simulink model "atrias_original"  (R2017a)
settings: Solver=ode45  StartTime=0.0  StopTime=sim_t  RelTol=1e-6  EnableMultiTasking=on
values from neighbouring files (symbols this model uses):
  N = grid_slice*1000    [createGrid.m]
  nm = fn_set_vnmc_params(sm, sample_time)    [kernel_scores_NM_mismatch.m]    (also in main_ATRIAS_cluster.m)
  nmc_BLCtrlPar = nmc.BLCtrlPar    [kernel_scores_NM_mismatch.m]    (also in main_ATRIAS_cluster.m)
  nmc_FPCtrlPar = nmc.FPCtrlPar    [kernel_scores_NM_mismatch.m]    (also in main_ATRIAS_cluster.m)
  nmc_LLCtrlPar = nmc.LLCtrlPar    [kernel_scores_NM_mismatch.m]    (also in main_ATRIAS_cluster.m)
  nmc_StCtrlPar = nmc.StCtrlPar    [kernel_scores_NM_mismatch.m]    (also in main_ATRIAS_cluster.m)
  nmc_SwCtrlPar = nmc.SwCtrlPar    [kernel_scores_NM_mismatch.m]    (also in main_ATRIAS_cluster.m)
  nmc_TrCtrlPar = nmc.TrCtrlPar    [kernel_scores_NM_mismatch.m]    (also in main_ATRIAS_cluster.m)
  nStep_switchCtrl = 10    [main_ATRIAS_cluster.m]
  nStep_thr = 1000    [createSimInitial.m]    (also in main_ATRIAS_cluster.m)
  rc_CtrlPar = [rc.k_placement, rc.T_step, rc.Cd, rc.kpt, rc.kdt, rc.desired_theta, rc.desired_z, rc.kpz, rc.kdz]    [kernel_scores_NM_mismatch.m]    (also in main_ATRIAS_cluster.m)
  sm = fn_set_MechParams(sm)    [kernel_scores_NM_mismatch.m]    (also in main_ATRIAS_cluster.m = fn_set_MechParams(sm,perturb))
  test_VNMC = 1    [createSimInitial.m]    (also in main_ATRIAS_cluster.m = 0)
undefined symbols (not defined in the file or in its folder): delta_phi_max, delta_phi_max_buffer, delta_phi_min, DiscIntNeverNeededParam, Discrete, idc, initial_dx_estimate, initial_dy_estimate, initial_dz_estimate, initial_z_estimate, kd_shin_max, kd_shin_min, kd_splay_max, kd_splay_min, kd_thigh_max, kd_thigh_min, kp_shin_max, kp_shin_min, kp_splay_max, kp_splay_min, kp_thigh_max, kp_thigh_min, mc, min_splay_angle, min_splay_buffer, phi_shin_max, phi_shin_max_buffer, phi_shin_min, phi_shin_min_buffer, phi_thigh_max, phi_thigh_max_buffer, phi_thigh_min, phi_thigh_min_buffer, rad, rc, s, sample_time, sgn, sim_d, t_friction, Time, X, Y, Z
libraries: sm_lib x202, nesl_utility x122, simulink x77, simulink_extras x24, fl_lib x16, mblibv1 x4, ctrlSharedLib x4, commnoisgen2 x1, dspswit3 x1
(part 5 of 17)

== system atrias_original/ATRIAS_sim/Mechanical System Layer/Torso ==
  Acceleration Sensor : sm_lib/Frames and Transforms/Transform Sensor  MeasurementFrame=NonRotatingFollower  SenseAngle=off  SenseAxis=off  SenseAngle1=off  SenseAngle2=off  SenseAngle3=off  SenseQ=off  SenseR=off  SenseOmegaX=off  SenseOmegaY=off  SenseOmegaZ=off  SenseOmega1=off  SenseOmega2=off  SenseOmega3=off  SenseQDot=off  SenseRDot=off  SenseAlphaX=off  SenseAlphaY=off  SenseAlphaZ=off  SenseAlpha1=off  SenseAlpha2=off  SenseAlpha3=off  SenseQDDot=off  SenseRDDot=off  SenseX=off  SenseY=off  SenseZ=off  SenseRad=off  SenseAzim=off  SenseDist=off  SenseInc=off  SenseXDot=off  SenseYDot=off  SenseZDot=off  SenseRadDot=off  SenseAzimDot=off  SenseDistDot=off  SenseIncDot=off  SenseXDDot=on  SenseYDDot=on  SenseZDDot=on  SenseRadDDot=off  SenseAzimDDot=off  SenseDistDDot=off  SenseIncDDot=off
  CS1 to CS2 : sm_lib/Frames and Transforms/Rigid Transform  TranslationMethod=Cartesian  TranslationStandardOffset=0  TranslationLengthUnit=m  TranslationStandardAxis=+Z  TranslationCartesianOffset=sm.torso_12  TranslationROffset=0  TranslationROffsetUnits=m  TranslationZOffset=0  TranslationZOffsetUnits=m  TranslationThetaOffset=0  TranslationThetaOffsetUnits=deg  RotationMethod=None  RotationAngleUnits=deg  RotationStandardAxis=+Z  RotationAngle=0  RotationArbitraryAxis=[0 0 1]  FollAlignAxisA=+X  BaseAlignAxisA=+Y  FollAlignAxisB=+Y  BaseAlignAxisB=+Z  RotationSequenceAxes=FollowerAxes  RotationSequence=XYX  RotationSequenceAngles=[0 0 0]  RotationSequenceAnglesUnits=deg  RotationMatrix=[1 0 0; 0 1 0; 0 0 1]
  Frame Data : Subsystem
  Hip Point to IMU : sm_lib/Frames and Transforms/Rigid Transform  TranslationMethod=Cartesian  TranslationStandardOffset=0  TranslationLengthUnit=m  TranslationStandardAxis=+Z  TranslationCartesianOffset=sm.d_pelvis_to_IMU  TranslationROffset=0  TranslationROffsetUnits=m  TranslationZOffset=0  TranslationZOffsetUnits=m  TranslationThetaOffset=0  TranslationThetaOffsetUnits=deg  RotationMethod=None  RotationAngleUnits=deg  RotationStandardAxis=+Z  RotationAngle=0  RotationArbitraryAxis=[0 0 1]  FollAlignAxisA=+X  BaseAlignAxisA=+Y  FollAlignAxisB=+Y  BaseAlignAxisB=+Z  RotationSequenceAxes=FollowerAxes  RotationSequence=XYX  RotationSequenceAngles=[0 0 0]  RotationSequenceAnglesUnits=deg  RotationMatrix=[1 0 0; 0 1 0; 0 0 1]
  Mux1 : Mux  Inputs=3
  Mux2 : Mux  Inputs=3
  Orientation Sensor : sm_lib/Frames and Transforms/Transform Sensor  MeasurementFrame=Base  SenseAngle=off  SenseAxis=off  SenseAngle1=off  SenseAngle2=off  SenseAngle3=off  SenseQ=off  SenseR=on  SenseOmegaX=off  SenseOmegaY=off  SenseOmegaZ=off  SenseOmega1=off  SenseOmega2=off  SenseOmega3=off  SenseQDot=off  SenseRDot=off  SenseAlphaX=off  SenseAlphaY=off  SenseAlphaZ=off  SenseAlpha1=off  SenseAlpha2=off  SenseAlpha3=off  SenseQDDot=off  SenseRDDot=off  SenseX=off  SenseY=off  SenseZ=off  SenseRad=off  SenseAzim=off  SenseDist=off  SenseInc=off  SenseXDot=off  SenseYDot=off  SenseZDot=off  SenseRadDot=off  SenseAzimDot=off  SenseDistDot=off  SenseIncDot=off  SenseXDDot=off  SenseYDDot=off  SenseZDDot=off  SenseRadDDot=off  SenseAzimDDot=off  SenseDistDDot=off  SenseIncDDot=off
  PS-Simulink Converter{1..3,8} (4 alike) : nesl_utility/PS-Simulink Converter  PhysicalDomain=network_engine_domain  SubClassName=ps_output  LeftPortType=input  RightPortType=output  PseudoPeriodic=off  Frequencies=[]  Unit=1  AffineConversion=off
  Rotation To Euler Angles : MATLAB Function  TreatAsAtomicUnit=on
  Solid : sm_lib/Body Elements/Solid  InertiaType=Custom  Mass=sm.m_torso  MassUnits=kg  CenterOfMass=sm.com_torso  CenterOfMassUnits=m  MomentsOfInertia=sm.i_torso_moments  MomentsOfInertiaUnits=kg*m^2  ProductsOfInertia=sm.i_torso_products  ProductsOfInertiaUnits=kg*m^2  DensityBased=on  Density=1000  DensityUnits=kg/(m^3)  DoExposeReferenceFrame=on  SerializedFrames=<Frames/>  GraphicType=FromGeometry  MarkerShape=Sphere  MarkerSize=10  MarkerSizeUnits=m  GraphicVisPropType=AdvancedVisualProperties  GraphicDiffuseColor=sm.torso_color_d  GraphicSpecularColor=[0.5 0.5 0.5 1.0]  GraphicAmbientColor=[sm.torso_color_d*0.5 1.0]  GraphicEmissiveColor=[0.0 0.0 0.0 1.0]  GraphicShininess=128  GraphicOpacity=1.0  GeometryShape=FromFile  RectangleSize=[1 1]  RectangleSizeUnits=m  BrickDimensions=[1 1 1]  BrickDimensionUnits=m  CylinderRadius=1  CylinderRadiusUnits=m  CylinderLength=1  CylinderLengthUnits=m  SphereRadius=1  SphereRadiusUnits=m  EllipsoidRadii=[1 1 1]  EllipsoidRadiiUnits=m  ExtrusionCrossSection=[1 1; -1 1; -1 -1; 1 -1]  ExtrusionCrossSectionUnits=m  ExtrusionLength=1  ExtrusionLengthUnits=m  PolygonNumSides=3  PolygonOuterRadius=1  PolygonOuterRadiusUnits=m  ExtGeomFileType=STL  ExtGeomFileName=../models/torso.stl  ExtGeomFileUnits=m  RevolutionCrossSection=[1 1; 1 -1; 2 -1; 2 1]  RevolutionCrossSectionUnits=m  RevolutionExtent=Full  RevolutionAngle=180  RevolutionAngleUnits=deg
  World Frame : sm_lib/Frames and Transforms/World Frame
  Yup to Zup Frame : sm_lib/Frames and Transforms/Rigid Transform  TranslationMethod=None  TranslationStandardOffset=0  TranslationLengthUnit=m  TranslationStandardAxis=+Z  TranslationCartesianOffset=0  TranslationROffset=0  TranslationROffsetUnits=m  TranslationZOffset=0  TranslationZOffsetUnits=m  TranslationThetaOffset=0  TranslationThetaOffsetUnits=deg  RotationMethod=AlignedAxes  RotationAngleUnits=deg  RotationStandardAxis=+Z  RotationAngle=0  RotationArbitraryAxis=[0 0 1]  FollAlignAxisA=+Z  BaseAlignAxisA=+Y  FollAlignAxisB=+X  BaseAlignAxisB=+X  RotationSequenceAxes=FollowerAxes  RotationSequence=XYX  RotationSequenceAngles=[0 0 0]  RotationSequenceAnglesUnits=deg  RotationMatrix=[1 0 0; 0 1 0; 0 0 1]
  CS1 : PMIOPort  Port=1  Side=Right
  CS2 : PMIOPort  Port=2  Side=Left
  CS3 : PMIOPort  Port=3  Side=Left
  IMU XYZ Accelerations [m/s^2] x3 : Outport
  IMU Orientation [rad x3] : Outport  Port=2
  wires:
  PS-Simulink Converter8/1 -> Mux1/1
  PS-Simulink Converter1/1 -> Mux1/2
  PS-Simulink Converter2/1 -> Mux1/3
  Mux1/1 -> IMU XYZ Accelerations [m/s^2] x3/1
  PS-Simulink Converter3/1 -> Rotation To Euler Angles/1(R)
  Rotation To Euler Angles/1(roll) -> Mux2/1
  Mux2/1 -> IMU Orientation [rad x3]/1
  Rotation To Euler Angles/3(yaw) -> Mux2/3
  Rotation To Euler Angles/2(pitch) -> Mux2/2
  connections:
  CS1 to CS2/LConn1 -- Frame Data/LConn1 -- CS1/RConn1 -- Solid/RConn1
  CS3/RConn1 -- CS2/RConn1 -- Hip Point to IMU/LConn1 -- CS1 to CS2/RConn1
  Orientation Sensor/RConn1 -- Acceleration Sensor/RConn1 -- Yup to Zup Frame/RConn1
  Hip Point to IMU/RConn1 -- Yup to Zup Frame/LConn1
  Acceleration Sensor/LConn1 -- World Frame/RConn1 -- Orientation Sensor/LConn1
  PS-Simulink Converter3/LConn1 -- Orientation Sensor/RConn2
  Acceleration Sensor/RConn2 -- PS-Simulink Converter8/LConn1
  Acceleration Sensor/RConn3 -- PS-Simulink Converter1/LConn1
  PS-Simulink Converter2/LConn1 -- Acceleration Sensor/RConn4

== system atrias_original/ATRIAS_sim/Mechanical System Layer/Winch ==
  note: Cable cannot push
  Compare To Constant1 : simulink/Logic and Bit Operations/Compare To Constant  relop===  const=-1  OutDataTypeStr=boolean  ZeroCross=off
  Constant1 : Constant  Value=sm.initial_winch_angle
  Constant2 : Constant  Value=0
  Desired Roll Velocity : Constant  Value=0
  Gain2 : Gain  Gain=sm.kp_winch
  Gain3 : Gain  Gain=sm.kd_winch
  PS-Simulink Converter : nesl_utility/PS-Simulink Converter  PhysicalDomain=network_engine_domain  SubClassName=ps_output  LeftPortType=input  RightPortType=output  PseudoPeriodic=off  Frequencies=[]  Unit=1  AffineConversion=off
  PS-Simulink Converter1 : nesl_utility/PS-Simulink Converter  PhysicalDomain=network_engine_domain  SubClassName=ps_output  LeftPortType=input  RightPortType=output  PseudoPeriodic=off  Frequencies=[]  Unit=1  AffineConversion=off
  Pitch Frame : sm_lib/Frames and Transforms/Rigid Transform  TranslationMethod=None  TranslationStandardOffset=0  TranslationLengthUnit=m  TranslationStandardAxis=+Z  TranslationCartesianOffset=[0 0 0]  TranslationROffset=0  TranslationROffsetUnits=m  TranslationZOffset=0  TranslationZOffsetUnits=m  TranslationThetaOffset=0  TranslationThetaOffsetUnits=deg  RotationMethod=AlignedAxes  RotationAngleUnits=rad  RotationStandardAxis=+Z  RotationAngle=0  RotationArbitraryAxis=[1 0 0]  FollAlignAxisA=-Z  BaseAlignAxisA=+X  FollAlignAxisB=+Y  BaseAlignAxisB=+Y  RotationSequenceAxes=FollowerAxes  RotationSequence=XYX  RotationSequenceAngles=[0 0 0]  RotationSequenceAnglesUnits=deg  RotationMatrix=[1 0 0; 0 1 0; 0 0 1]
  Roll Frame : sm_lib/Frames and Transforms/Rigid Transform  TranslationMethod=None  TranslationStandardOffset=0  TranslationLengthUnit=m  TranslationStandardAxis=+Z  TranslationCartesianOffset=[0 0 0]  TranslationROffset=0  TranslationROffsetUnits=m  TranslationZOffset=0  TranslationZOffsetUnits=m  TranslationThetaOffset=0  TranslationThetaOffsetUnits=deg  RotationMethod=AlignedAxes  RotationAngleUnits=rad  RotationStandardAxis=+Z  RotationAngle=0  RotationArbitraryAxis=[1 0 0]  FollAlignAxisA=+X  BaseAlignAxisA=-Z  FollAlignAxisB=+Y  BaseAlignAxisB=+Y  RotationSequenceAxes=FollowerAxes  RotationSequence=XYX  RotationSequenceAngles=[0 0 0]  RotationSequenceAnglesUnits=deg  RotationMatrix=[1 0 0; 0 1 0; 0 0 1]
  Roll Joint : sm_lib/Joints/Revolute Joint  SenseConstraintForce=off  SenseConstraintForceX=off  SenseConstraintForceY=off  SenseConstraintForceZ=off  SenseConstraintTorque=off  SenseConstraintTorqueX=off  SenseConstraintTorqueY=off  SenseConstraintTorqueZ=off  SenseTotalForce=off  SenseTotalForceX=off  SenseTotalForceY=off  SenseTotalForceZ=off  SenseTotalTorque=off  SenseTotalTorqueX=off  SenseTotalTorqueY=off  SenseTotalTorqueZ=off  CompositeWrenchDir=FollowerOnBase  CompositeWrenchFrame=BaseFrame  EquilibriumPosition=0  EquilibriumPositionUnits=deg  SpringStiffness=0  SpringStiffnessUnits=N*m/deg  DampingCoefficient=0  DampingCoefficientUnits=N*m/(deg/s)  TorqueActuationMode=InputTorque  MotionActuationMode=ComputedMotion  SensePosition=on  SenseVelocity=on  SenseAcceleration=off  SenseTorqueForce=off  PositionTargetSpecify=on  PositionTargetPriority=High  PositionTargetValue=sm.initial_boom_roll  PositionTargetValueUnits=rad  VelocityTargetSpecify=off  VelocityTargetPriority=High  VelocityTargetValue=0  VelocityTargetValueUnits=deg/s
  Sign1 : Signum  ZeroCross=off
  Simulink-PS Converter : nesl_utility/Simulink-PS Converter  PhysicalDomain=network_engine_domain  SubClassName=ps_input  LeftPortType=input  RightPortType=output  PseudoPeriodic=off  Frequencies=[]  NoiseDistribution=none  NoiseParameters=[]  Unit=1  AffineConversion=off  FilteringAndDerivatives=zero  SimscapeFilterOrder=1  InputFilterTimeConstant=0.001  UdotUserProvided=1
  Sum : Sum  Inputs=+-|
  Sum1 : Sum  Inputs=+|+
  Sum3 : Sum  Inputs=+-|
  Switch : Switch  Threshold=1
  Boom : PMIOPort  Port=1  Side=Right
  Yaw Shaft : PMIOPort  Port=2  Side=Right
  Boom Roll [rad] : Outport
  wires:
  Sum/1 -> Gain2/1
  Sum1/1 -> Switch/3, Sign1/1
  Sign1/1 -> Compare To Constant1/1
  Constant2/1 -> Switch/1
  Compare To Constant1/1 -> Switch/2
  Switch/1 -> Simulink-PS Converter/1
  PS-Simulink Converter/1 -> Boom Roll [rad]/1, Sum/2
  PS-Simulink Converter1/1 -> Sum3/2
  Desired Roll Velocity/1 -> Sum3/1
  Sum3/1 -> Gain3/1
  Gain2/1 -> Sum1/1
  Gain3/1 -> Sum1/2
  Constant1/1 -> Sum/1
  connections:
  Roll Frame/RConn1 -- Roll Joint/LConn1
  Roll Frame/LConn1 -- Yaw Shaft/RConn1
  Boom/RConn1 -- Pitch Frame/RConn1
  Pitch Frame/LConn1 -- Roll Joint/RConn1
  Roll Joint/LConn2 -- Simulink-PS Converter/RConn1
  PS-Simulink Converter/LConn1 -- Roll Joint/RConn2
  PS-Simulink Converter1/LConn1 -- Roll Joint/RConn3

== system atrias_original/ATRIAS_sim/Mechanical System Layer/Yaw Joint ==
  PS-Simulink Converter3 : nesl_utility/PS-Simulink Converter  PhysicalDomain=network_engine_domain  SubClassName=ps_output  LeftPortType=input  RightPortType=output  PseudoPeriodic=off  Frequencies=[]  Unit=1  AffineConversion=off
  Roll Frame : sm_lib/Frames and Transforms/Rigid Transform  TranslationMethod=None  TranslationStandardOffset=0  TranslationLengthUnit=m  TranslationStandardAxis=+Z  TranslationCartesianOffset=[0 0 0]  TranslationROffset=0  TranslationROffsetUnits=m  TranslationZOffset=0  TranslationZOffsetUnits=m  TranslationThetaOffset=0  TranslationThetaOffsetUnits=deg  RotationMethod=AlignedAxes  RotationAngleUnits=rad  RotationStandardAxis=+Z  RotationAngle=0  RotationArbitraryAxis=[1 0 0]  FollAlignAxisA=+Z  BaseAlignAxisA=+Y  FollAlignAxisB=+X  BaseAlignAxisB=+X  RotationSequenceAxes=FollowerAxes  RotationSequence=XYX  RotationSequenceAngles=[0 0 0]  RotationSequenceAnglesUnits=deg  RotationMatrix=[1 0 0; 0 1 0; 0 0 1]
  Yaw Frame : sm_lib/Frames and Transforms/Rigid Transform  TranslationMethod=None  TranslationStandardOffset=0  TranslationLengthUnit=m  TranslationStandardAxis=+Z  TranslationCartesianOffset=[0 0 0]  TranslationROffset=0  TranslationROffsetUnits=m  TranslationZOffset=0  TranslationZOffsetUnits=m  TranslationThetaOffset=0  TranslationThetaOffsetUnits=deg  RotationMethod=AlignedAxes  RotationAngleUnits=rad  RotationStandardAxis=+Z  RotationAngle=0  RotationArbitraryAxis=[1 0 0]  FollAlignAxisA=+Y  BaseAlignAxisA=+Z  FollAlignAxisB=+X  BaseAlignAxisB=+X  RotationSequenceAxes=FollowerAxes  RotationSequence=XYX  RotationSequenceAngles=[0 0 0]  RotationSequenceAnglesUnits=deg  RotationMatrix=[1 0 0; 0 1 0; 0 0 1]
  Yaw Joint : sm_lib/Joints/Revolute Joint  SenseConstraintForce=off  SenseConstraintForceX=off  SenseConstraintForceY=off  SenseConstraintForceZ=off  SenseConstraintTorque=off  SenseConstraintTorqueX=off  SenseConstraintTorqueY=off  SenseConstraintTorqueZ=off  SenseTotalForce=off  SenseTotalForceX=off  SenseTotalForceY=off  SenseTotalForceZ=off  SenseTotalTorque=off  SenseTotalTorqueX=off  SenseTotalTorqueY=off  SenseTotalTorqueZ=off  CompositeWrenchDir=FollowerOnBase  CompositeWrenchFrame=BaseFrame  EquilibriumPosition=0  EquilibriumPositionUnits=deg  SpringStiffness=0  SpringStiffnessUnits=N*m/deg  DampingCoefficient=0  DampingCoefficientUnits=N*m/(deg/s)  TorqueActuationMode=NoTorque  MotionActuationMode=ComputedMotion  SensePosition=on  SenseVelocity=off  SenseAcceleration=off  SenseTorqueForce=off  PositionTargetSpecify=on  PositionTargetPriority=High  PositionTargetValue=sm.initial_boom_yaw  PositionTargetValueUnits=rad  VelocityTargetSpecify=on  VelocityTargetPriority=High  VelocityTargetValue=sm.initial_boom_yaw_velocity  VelocityTargetValueUnits=rad/s
  Yaw Shaft : PMIOPort  Port=1  Side=Right
  Base : PMIOPort  Port=2  Side=Left
  Yaw [rad] : Outport
  wires:
  PS-Simulink Converter3/1 -> Yaw [rad]/1
  connections:
  Yaw Frame/LConn1 -- Base/RConn1
  Yaw Joint/LConn1 -- Yaw Frame/RConn1
  Roll Frame/LConn1 -- Yaw Joint/RConn1
  Roll Frame/RConn1 -- Yaw Shaft/RConn1
  PS-Simulink Converter3/LConn1 -- Yaw Joint/RConn2

== system atrias_original/ATRIAS_sim/Mechanical System Layer/Yaw Shaft ==
  CS1 to CS2 : sm_lib/Frames and Transforms/Rigid Transform  TranslationMethod=Cartesian  TranslationStandardOffset=0  TranslationLengthUnit=m  TranslationStandardAxis=+Z  TranslationCartesianOffset=sm.yshaft_12  TranslationROffset=0  TranslationROffsetUnits=m  TranslationZOffset=0  TranslationZOffsetUnits=m  TranslationThetaOffset=0  TranslationThetaOffsetUnits=deg  RotationMethod=None  RotationAngleUnits=deg  RotationStandardAxis=+Z  RotationAngle=0  RotationArbitraryAxis=[0 0 1]  FollAlignAxisA=+X  BaseAlignAxisA=+Y  FollAlignAxisB=+Y  BaseAlignAxisB=+Z  RotationSequenceAxes=FollowerAxes  RotationSequence=XYX  RotationSequenceAngles=[0 0 0]  RotationSequenceAnglesUnits=deg  RotationMatrix=[1 0 0; 0 1 0; 0 0 1]
  External Boom Camera : sm_lib/Frames and Transforms/Rigid Transform  TranslationMethod=Cartesian  TranslationStandardOffset=0  TranslationLengthUnit=m  TranslationStandardAxis=+Z  TranslationCartesianOffset=[0 0 -4.5]  TranslationROffset=0  TranslationROffsetUnits=m  TranslationZOffset=0  TranslationZOffsetUnits=m  TranslationThetaOffset=0  TranslationThetaOffsetUnits=deg  RotationMethod=None  RotationAngleUnits=deg  RotationStandardAxis=+Z  RotationAngle=0  RotationArbitraryAxis=[0 0 1]  FollAlignAxisA=+X  BaseAlignAxisA=+Y  FollAlignAxisB=+Y  BaseAlignAxisB=+Z  RotationSequenceAxes=FollowerAxes  RotationSequence=XYX  RotationSequenceAngles=[0 0 0]  RotationSequenceAnglesUnits=deg  RotationMatrix=[1 0 0; 0 1 0; 0 0 1]
  Frame Data : Subsystem
  Solid : sm_lib/Body Elements/Solid  InertiaType=Custom  Mass=sm.m_yshaft  MassUnits=kg  CenterOfMass=sm.com_yshaft  CenterOfMassUnits=m  MomentsOfInertia=sm.i_yshaft_moments  MomentsOfInertiaUnits=kg*m^2  ProductsOfInertia=sm.i_yshaft_products  ProductsOfInertiaUnits=kg*m^2  DensityBased=on  Density=1000  DensityUnits=kg/(m^3)  DoExposeReferenceFrame=on  SerializedFrames=<Frames/>  GraphicType=FromGeometry  MarkerShape=Sphere  MarkerSize=10  MarkerSizeUnits=m  GraphicVisPropType=AdvancedVisualProperties  GraphicDiffuseColor=sm.yshaft_color_d  GraphicSpecularColor=[0.5 0.5 0.5 1.0]  GraphicAmbientColor=[sm.yshaft_color_d*0.5 1.0]  GraphicEmissiveColor=[0.0 0.0 0.0 1.0]  GraphicShininess=128  GraphicOpacity=1.0  GeometryShape=FromFile  RectangleSize=[1 1]  RectangleSizeUnits=m  BrickDimensions=[1 1 1]  BrickDimensionUnits=m  CylinderRadius=1  CylinderRadiusUnits=m  CylinderLength=1  CylinderLengthUnits=m  SphereRadius=1  SphereRadiusUnits=m  EllipsoidRadii=[1 1 1]  EllipsoidRadiiUnits=m  ExtrusionCrossSection=[1 1; -1 1; -1 -1; 1 -1]  ExtrusionCrossSectionUnits=m  ExtrusionLength=1  ExtrusionLengthUnits=m  PolygonNumSides=3  PolygonOuterRadius=1  PolygonOuterRadiusUnits=m  ExtGeomFileType=STL  ExtGeomFileName=../models/boom_yaw.stl  ExtGeomFileUnits=m  RevolutionCrossSection=[1 1; 1 -1; 2 -1; 2 1]  RevolutionCrossSectionUnits=m  RevolutionExtent=Full  RevolutionAngle=180  RevolutionAngleUnits=deg
  CS1 : PMIOPort  Port=1  Side=Left
  CS2 : PMIOPort  Port=2  Side=Right
  connections:
  CS2/RConn1 -- External Boom Camera/LConn1 -- CS1 to CS2/RConn1
  CS1/RConn1 -- CS1 to CS2/LConn1 -- Solid/RConn1 -- Frame Data/LConn1

== system atrias_original/Actuator Control Layer/SEA Controller (Torque)/Desired Torque Derivative ==
  Signal x4 : Inport
  Reset [1/0] x4 : Inport  Port=2
  Demux : Demux
  Demux1 : Demux
  Gain1 : Gain  Gain=1/sample_time
  Logical Operator : Logic  Operator=NOT  AllPortsSameDT=off  OutDataTypeStr=boolean
  Mux : Mux
  Product : Product
  difference : simulink/Discrete/Difference  ICPrevInput=0.0  InputProcessing=Inherited  OutMin=[]  OutMax=[]  OutDataType=fixdt(1, 16)  OutScaling=2^-10  DoSatur=off
  two_pole_filter{,1..3} (4 alike) : DiscreteTransferFcn  Numerator=[mc.A_lpf_dtau 0 0]  Denominator=[1 mc.B1_lpf_dtau mc.B2_lpf_dtau]  ExternalReset=Rising  SampleTime=sample_time
      settings: InputPortMap=u0,r7
  Derivative x4 : Outport
  wires:
  Demux/1 -> two_pole_filter/1
  difference/1 -> Product/1
  Mux/1 -> Derivative x4/1
  Signal x4/1 -> Gain1/1
  Gain1/1 -> difference/1
  Logical Operator/1 -> Product/2
  Reset [1/0] x4/1 -> Demux1/1, Logical Operator/1
  two_pole_filter/1 -> Mux/1
  Product/1 -> Demux/1
  two_pole_filter1/1 -> Mux/2
  two_pole_filter2/1 -> Mux/3
  two_pole_filter3/1 -> Mux/4
  Demux/2 -> two_pole_filter1/1
  Demux/3 -> two_pole_filter2/1
  Demux/4 -> two_pole_filter3/1
  Demux1/1 -> two_pole_filter/2
  Demux1/2 -> two_pole_filter1/2
  Demux1/3 -> two_pole_filter2/2
  Demux1/4 -> two_pole_filter3/2

== system atrias_original/control/Data/Subsystem ==
  In : Inport
  Enable : EnablePort
  Out1 : Outport
  wires:
  In/1 -> Out1/1

== system atrias_original/control/Data/Subsystem1 ==
  In1 : Inport
  Enable : EnablePort
  Out1 : Outport
  wires:
  In1/1 -> Out1/1

== system atrias_original/control/Data/state at switch ==
  xTorso : Inport
  Trigger : TriggerPort  VariantControl=Variant  ZeroCross=off
  To Current Workspace2 : ToWorkspace  VariableName=simout_xTorso_switch  SaveFormat=Structure With Time  SampleTime=-1
      settings: MaxDataPoints=1
  wires:
  xTorso/1 -> To Current Workspace2/1

== system atrias_original/control/RC control/Atrias Swing control ==
  note: Convert to
      | four-bar angles
  note: Position control the
      | individual four bar segments
  X COM from Secondary Foot Desired [m m/s m/s^2] : Inport
  Y COM  from Secondary Foot Desired [m m/s m/s^2] : Inport  Port=2
  Z COM  from Secondary Foot Desired [m m/s m/s^2] : Inport  Port=3
  Secondary Front Gear [rad rad/s] : Inport  Port=4
  Secondary Back Gear [rad rad/s] : Inport  Port=5
  Right or Left Stance [1 or 0] : Inport  Port=6
  Secondary Leg Roll [rad rad/s] : Inport  Port=7
  Secondary Leg Length [m m/s] : Inport  Port=8
  Secondary Leg Angle [rad rad/s] : Inport  Port=9
  Torso Pitch [rad rad/s] : Inport  Port=10
  Torso Roll [rad rad/s] : Inport  Port=11
  Pelvis to COM Position [m] x3 : Inport  Port=12
  Pelvis to COM Velocity [m/s] x3 : Inport  Port=13
  Avoid Hitting Mechanical Limits : MATLAB Function  TreatAsAtomicUnit=on
  Back/Front PD : Subsystem
  "Convert COM Position to Joint Angles + Leg Length " : MATLAB Function  TreatAsAtomicUnit=on
  Demux4 : Demux  Outputs=2
  Demux5 : Demux  Outputs=2
  Demux6 : Demux  Outputs=6
  Mux{3..6,8,11} (6 alike) : Mux  Inputs=2
  Virtual Leg to Four Bar : MATLAB Function  TreatAsAtomicUnit=on
  Back Front Motor Torques [Nm Nm] : Outport
  Desired Swing Beta [rad rad/s] : Outport  Port=2
  wires:
  Virtual Leg to Four Bar/5(dfront) -> Avoid Hitting Mechanical Limits/5(dfront_desired)
  Y COM  from Secondary Foot Desired [m m/s m/s^2]/1 -> "Convert COM Position to Joint Angles + Leg Length "/2(Y_star)
  Mux8/1 -> Demux6/1
  "Convert COM Position to Joint Angles + Leg Length "/1(desired_leg_length) -> Mux8/1
  X COM from Secondary Foot Desired [m m/s m/s^2]/1 -> "Convert COM Position to Joint Angles + Leg Length "/1(X_star)
  Secondary Leg Length [m m/s]/1 -> "Convert COM Position to Joint Angles + Leg Length "/11(leg_length)
  "Convert COM Position to Joint Angles + Leg Length "/3(desired_beta) -> Desired Swing Beta [rad rad/s]/1  "lateral motor angle"
  "Convert COM Position to Joint Angles + Leg Length "/2(desired_alpha) -> Mux8/2
  Secondary Leg Angle [rad rad/s]/1 -> "Convert COM Position to Joint Angles + Leg Length "/9(sagittal_angle)
  Secondary Leg Roll [rad rad/s]/1 -> "Convert COM Position to Joint Angles + Leg Length "/10(lateral_angle)  "swing hip angle (lateral)"
  Right or Left Stance [1 or 0]/1 -> "Convert COM Position to Joint Angles + Leg Length "/4(right_left)
  Torso Roll [rad rad/s]/1 -> "Convert COM Position to Joint Angles + Leg Length "/7(roll)
  Torso Pitch [rad rad/s]/1 -> "Convert COM Position to Joint Angles + Leg Length "/8(pitch)
  Virtual Leg to Four Bar/1(back) -> Avoid Hitting Mechanical Limits/1(back_desired)
  Demux4/2 -> Mux11/2
  Demux6/5 -> Virtual Leg to Four Bar/5(dphi)
  Virtual Leg to Four Bar/4(front) -> Avoid Hitting Mechanical Limits/4(front_desired)
  Demux6/6 -> Virtual Leg to Four Bar/6(ddphi)
  Demux6/3 -> Virtual Leg to Four Bar/3(ddl_leg)
  Demux6/2 -> Virtual Leg to Four Bar/2(dl_leg)
  Virtual Leg to Four Bar/3(ddback) -> Avoid Hitting Mechanical Limits/3(ddback_desired)
  Virtual Leg to Four Bar/6(ddfront) -> Avoid Hitting Mechanical Limits/6(ddfront_desired)
  Mux11/1 -> Back/Front PD/5(Measured Velocity [rad/s] [back front])
  Virtual Leg to Four Bar/2(dback) -> Avoid Hitting Mechanical Limits/2(dback_desired)
  Demux6/4 -> Virtual Leg to Four Bar/4(phi)
  Demux6/1 -> Virtual Leg to Four Bar/1(l_leg)
  Back/Front PD/1(Commanded Torque [Nm] [back front]) -> Back Front Motor Torques [Nm Nm]/1
  Secondary Back Gear [rad rad/s]/1 -> Demux5/1
  Demux5/1 -> Mux6/1
  Z COM  from Secondary Foot Desired [m m/s m/s^2]/1 -> "Convert COM Position to Joint Angles + Leg Length "/3(Z_star)
  Mux4/1 -> Back/Front PD/2(Desired Velocity [rad/s] [back front])
  Secondary Front Gear [rad rad/s]/1 -> Demux4/1
  Demux5/2 -> Mux11/1
  Avoid Hitting Mechanical Limits/3(dback_cmd) -> Mux4/1
  Mux5/1 -> Back/Front PD/3(Desired Acceleration [rad/s^2] [back front])
  Mux3/1 -> Back/Front PD/1(Desired Position [rad] [back front])
  Mux6/1 -> Back/Front PD/4(Measured Position [rad] [back front])
  Avoid Hitting Mechanical Limits/6(ddfront_cmd) -> Mux5/2
  Avoid Hitting Mechanical Limits/5(ddback_cmd) -> Mux5/1
  Avoid Hitting Mechanical Limits/2(front_cmd) -> Mux3/2
  Avoid Hitting Mechanical Limits/4(dfront_cmd) -> Mux4/2
  Avoid Hitting Mechanical Limits/1(back_cmd) -> Mux3/1
  Demux4/1 -> Mux6/2
  Pelvis to COM Position [m] x3/1 -> "Convert COM Position to Joint Angles + Leg Length "/5(com_pelvis_body)
  Pelvis to COM Velocity [m/s] x3/1 -> "Convert COM Position to Joint Angles + Leg Length "/6(dcom_pelvis_body)

== system atrias_original/control/RC control/Enabled Subsystem1 ==
  In1 : Inport
  Enable : EnablePort
  Out1 : Outport
  wires:
  In1/1 -> Out1/1

== system atrias_original/control/RC control/Estimate Angular Accelerations2 ==
  Angular Velocities [rad/s] x3 : Inport
  Enabled : Inport  Port=2
  Detect Change : simulink/Logic and Bit Operations/Detect Change  vinit=0  InputProcessing=Inherited  OutDataTypeStr=boolean
  Difference : simulink/Discrete/Difference  ICPrevInput=0.0  InputProcessing=Inherited  OutMin=[]  OutMax=[]  OutDataType=fixdt(1, 16)  OutScaling=2^-10  DoSatur=off
  Gain : Gain  Gain=1/sample_time
  IMU Two Pole Filter1 : DiscreteTransferFcn  Numerator=[mc.A_lpf_imu 0 0]  Denominator=[1 mc.B1_lpf_imu mc.B2_lpf_imu]  SampleTime=sample_time
  Logical Operator5 : Logic  Operator=NOT  AllPortsSameDT=off  OutDataTypeStr=boolean
  Product : Product
  Angular Accelerations [rad/s^2] x3 : Outport
  wires:
  Enabled/1 -> Detect Change/1
  Logical Operator5/1 -> Product/2
  Angular Velocities [rad/s] x3/1 -> Difference/1
  Gain/1 -> Product/1
  Difference/1 -> Gain/1
  Detect Change/1 -> Logical Operator5/1
  Product/1 -> IMU Two Pole Filter1/1
  IMU Two Pole Filter1/1 -> Angular Accelerations [rad/s^2] x3/1

== system atrias_original/control/RC control/Estimate Angular Accelerations3 ==
  Angular Velocities [rad/s] x2 : Inport
  Enabled : Inport  Port=2
  Detect Change : simulink/Logic and Bit Operations/Detect Change  vinit=0  InputProcessing=Inherited  OutDataTypeStr=boolean
  Difference : simulink/Discrete/Difference  ICPrevInput=0.0  InputProcessing=Inherited  OutMin=[]  OutMax=[]  OutDataType=fixdt(1, 16)  OutScaling=2^-10  DoSatur=off
  Gain : Gain  Gain=1/sample_time
  Lateral Angle Two Pole Filter1 : DiscreteTransferFcn  Numerator=[mc.A_lpf_lateral_angle 0 0]  Denominator=[1 mc.B1_lpf_lateral_angle mc.B2_lpf_lateral_angle]  SampleTime=sample_time
  Logical Operator5 : Logic  Operator=NOT  AllPortsSameDT=off  OutDataTypeStr=boolean
  Product : Product
  Angular Accelerations [rad/s^2] x2 : Outport
  wires:
  Detect Change/1 -> Logical Operator5/1
  Difference/1 -> Gain/1
  Gain/1 -> Product/1
  Angular Velocities [rad/s] x2/1 -> Difference/1
  Logical Operator5/1 -> Product/2
  Enabled/1 -> Detect Change/1
  Product/1 -> Lateral Angle Two Pole Filter1/1
  Lateral Angle Two Pole Filter1/1 -> Angular Accelerations [rad/s^2] x2/1

== system atrias_original/control/RC control/Fz_commanded ==
  measured_z : Inport
  measured_zd : Inport  Port=2
  desired_z : Inport  Port=3
  "Primary Measured Vertical [N}" : Inport  Port=4
  COM XYZ Acceleration [m/s^2] x3 : Inport  Port=5
  kpz : Inport  Port=6
  kdz : Inport  Port=7
  Clamp2 : Saturate  UpperLimit=inf  LowerLimit=0
      settings: AttributesFormatString=Top: %<UpperLimit>\nBottom: %<LowerLimit>
  Clamp3 : Saturate  UpperLimit=inf  LowerLimit=1
      settings: AttributesFormatString=Top: %<UpperLimit>\nBottom: %<LowerLimit>
  Clamp4 : Saturate  UpperLimit=1  LowerLimit=0
      settings: AttributesFormatString=Top: %<UpperLimit>\nBottom: %<LowerLimit>
  Compute Forces1 : Subsystem
  Constant1 : Constant  Commented=on  Value=0.87
  Constant2 : Constant  Commented=on
  Constant3 : Constant
  Constant6 : Constant  Value=mc.m_total_real*mc.g
  Constant7 : Constant  Value=0
  Divide : Product  Inputs=**
  Divide1 : Product  Inputs=*/
  Fcn : Fcn  Expr=1-u
  From82 : From  Commented=on  GotoTag=RightLeft
  Fz : Scope
  Fz Factor : Scope
  Gain8 : Gain  Gain=1/(2*mc.m_total_real*mc.g)
  Mux : Mux  Inputs=2
  Mux35 : Mux  Inputs=2
  Saturation : Saturate  UpperLimit=Inf  LowerLimit=0.2*mc.m_total_real*mc.g
  Selector14 : Selector  InputPortWidth=3  IndexOptions=Index vector (dialog)  Indices=[3]  OutputSizes=1
  Sum1 : Sum  Inputs=|++
  Sum2 : Sum  Inputs=+|+
  Sum3 : Sum  Inputs=+-|
  Sum4 : Sum  Inputs=+++
  Sum6 : Sum  Inputs=+-|
  Switch4 : Switch  Commented=on  Criteria=u2 ~= 0
  multiply : Product  Inputs=**
  multiply1 : Product  Inputs=**
  times : Product  Inputs=**
  times1 : Product  Inputs=**
  z tracking : Scope  NumInputPorts=2
  Fz_commanded : Outport
  wires:
  desired_z/1 -> z tracking/1, Sum3/1
  Saturation/1 -> Mux/2, Fz_commanded/1
  measured_zd/1 -> Sum6/2
  Sum6/1 -> multiply1/1
  Constant7/1 -> Sum6/1
  Sum3/1 -> multiply/1
  measured_z/1 -> z tracking/2, Sum3/2
  Constant6/1 -> Sum4/3
  multiply/1 -> Sum4/1
  multiply1/1 -> Sum4/2
  [GRF_Lz] -> Sum1/1
  [GRF_Rz] -> Sum1/2
  Mux/1 -> Fz/1
  Sum1/1 -> Mux/1
  Divide/1 -> Saturation/1
  Sum4/1 -> Divide/1
  Constant1/1 -> Switch4/3
  Constant2/1 -> Switch4/1
  From82/1 -> Switch4/2
  [GRFfromAccelerometer] -> Selector14/1
  "Primary Measured Vertical [N}"/1 -> Clamp2/1
  Selector14/1 -> Clamp3/1
  Clamp3/1 -> Divide1/2, Gain8/1
  Divide1/1 -> Mux35/1, times/1
  Sum2/1 -> [FzFactor], Mux35/2
  Gain8/1 -> Clamp4/1
  Clamp4/1 -> times/2, Fcn/1
  times/1 -> Sum2/1
  Fcn/1 -> times1/1
  Constant3/1 -> times1/2
  times1/1 -> Sum2/2
  Mux35/1 -> Fz Factor/1
  Clamp2/1 -> Divide1/1
  COM XYZ Acceleration [m/s^2] x3/1 -> Compute Forces1/1(XYZ Acceleration)
  Compute Forces1/1(XYZ Force) -> [GRFfromAccelerometer]
  [FzFactor] -> Divide/2
  kpz/1 -> multiply/2
  kdz/1 -> multiply1/2

== system atrias_original/control/RC control/Inverse Dynamics 2D ==
  Desired Vertical GRF [N] : Inport
  Desired Forward GRF [N] : Inport  Port=2
  Leg Length [m m/s] : Inport  Port=3
  Leg Angle [rad rad/s] : Inport  Port=4
  Torso Pitch [rad rad/s] : Inport  Port=5
  Primary w [m] : Inport  Port=6
  Constant2 : Constant  Value=0
  Demux5 : Demux  Outputs=2
  Leg Force-Torque Distribution : Subsystem
  Spring Torques : Selector  InputPortWidth=7  IndexOptions=Index vector (dialog)  Indices=[6 7]  OutputSizes=1
  target_GRF_inverse_dynamics : MATLAB Function  TreatAsAtomicUnit=on
  Leg Force [N] : Outport
  Leg Torque [Nm] : Outport  Port=2
  wires:
  Desired Vertical GRF [N]/1 -> target_GRF_inverse_dynamics/2(GRFz)
  Desired Forward GRF [N]/1 -> target_GRF_inverse_dynamics/1(GRFx)
  Leg Length [m m/s]/1 -> target_GRF_inverse_dynamics/5(l_leg)
  Constant2/1 -> target_GRF_inverse_dynamics/7(tau_rotor_f), target_GRF_inverse_dynamics/8(tau_rotor_b)
  target_GRF_inverse_dynamics/1(z) -> Spring Torques/1
  Demux5/2 -> Leg Force-Torque Distribution/2(Back Spring Torque [Nm])
  Demux5/1 -> Leg Force-Torque Distribution/1(Front Spring Torque [Nm])
  Spring Torques/1 -> Demux5/1
  Primary w [m]/1 -> Leg Force-Torque Distribution/3(w [m]), target_GRF_inverse_dynamics/6(w)
  Leg Force-Torque Distribution/2(Leg Torque [Nm]) -> Leg Torque [Nm]/1
  Torso Pitch [rad rad/s]/1 -> target_GRF_inverse_dynamics/3(theta)
  Leg Angle [rad rad/s]/1 -> target_GRF_inverse_dynamics/4(phi)
  Leg Force-Torque Distribution/1(Leg Force [N]) -> Leg Force [N]/1

== system atrias_original/control/RC control/Primary Secondary Leg Swap ==
  note: q Order:
      |
      | backJointR
      | backGearR
      | frontJointR
      | frontGearR
      |
      | backJointL
      | backGearL
      | frontJointL
      | frontGearL
      |
      | latR
      | latL
      |
      | boomRoll
      | boomYaw
      | boomPitch
  Entering Stance [1/0] : Inport
  R Leg Angle [rad rad/s] : Inport  Port=2
  R Leg Length [m m/s] : Inport  Port=3
  R Leg w [m] : Inport  Port=4
  R Back Joint [rad rad/s] : Inport  Port=5
  R Back Gear [rad rad/s] : Inport  Port=6
  R Front Joint [rad rad/s] : Inport  Port=7
  R Front Gear [rad rad/s] : Inport  Port=8
  L Leg Angle [rad rad/s] : Inport  Port=9
  L Leg Length [m m/s] : Inport  Port=10
  L Leg w [m] : Inport  Port=11
  L Back Joint [rad rad/s] : Inport  Port=12
  L Back Gear [rad rad/s] : Inport  Port=13
  L Front Joint [rad rad/s] : Inport  Port=14
  L Front Gear [rad rad/s] : Inport  Port=15
  Primary Force/Position Control [1/0] : Inport  Port=16
  Primary Back/Front SEA Torque [Nm Nm] : Inport  Port=17
  Primary Back/Front Motor Torque [Nm Nm] : Inport  Port=18
  Secondary Force/Position Control [1/0] : Inport  Port=19
  Secondary Back/Front SEA Torque [Nm Nm] : Inport  Port=20
  Secondary Back/Front Motor Torque [Nm Nm] : Inport  Port=21
  "Right Leg Roll [rad, rad/s]" : Inport  Port=22
  "Left Leg Roll [rad, rad/s]" : Inport  Port=23
  System Time [s] : Inport  Port=24
  Bus Creator : BusCreator  Inputs=22
  Bus Creator1 : BusCreator  Inputs=22
  Bus Selector : BusSelector  OutputSignals=signal1,signal2,signal3,signal4,signal5,signal6,signal7,signal8,signal9,signal10,signal11,signal12,signal13,signal14,signal15,signal16,signal17,signal18,signal19,signal20,signal21,signal22
  Enabled Subsystem : Subsystem  TreatAsAtomicUnit=on
  Manual Switch : ManualSwitch
  Right Left Primary : Scope  NumInputPorts=2
  Select Leg : Constant  OutDataTypeStr=boolean
  Sum5 : Sum  Inputs=|-+
  Switch6 : Switch  Criteria=u2 ~= 0  OutDataTypeStr=Inherit: Inherit via back propagation  ZeroCross=off
  ToggleRightLeftLeg : MATLAB Function  TreatAsAtomicUnit=on
      settings: MinAlgLoopOccurrences=on
  Unit Delay : UnitDelay  InitialCondition=rc.manual_leg_selection  SampleTime=sample_time
  Right/Left Primary [1/0] : Outport
  Primary Leg Angle [rad rad/s] : Outport  Port=2
  Primary Leg Length [m m/s] : Outport  Port=3
  Primary Leg w [m] : Outport  Port=4
  Primary Back Joint [rad rad/s] : Outport  Port=5
  Primary Back Gear [rad rad/s] : Outport  Port=6
  Primary Front Joint [rad rad/s] : Outport  Port=7
  Primary Front Gear [rad rad/s] : Outport  Port=8
  Secondary Leg Angle [rad rad/s] : Outport  Port=9
  Secondary Leg Length [rad rad/s] : Outport  Port=10
  Secondary Leg w [m] : Outport  Port=11
  Secondary Back Joint [rad rad/s] : Outport  Port=12
  Secondary Back Gear [rad rad/s] : Outport  Port=13
  Secondary Front Joint [rad rad/s] : Outport  Port=14
  Secondary Front Gear [rad rad/s] : Outport  Port=15
  R Force/Position Control [1/0] : Outport  Port=16
  R Back/Front SEA Torque [Nm Nm] : Outport  Port=17
  R Back/Front Motor Torque [Nm Nm] : Outport  Port=18
  L Force/Position Control [1/0] : Outport  Port=19
  L Back/Front SEA Torque [Nm Nm] : Outport  Port=20
  L Back/Front Motor Torque [Nm Nm] : Outport  Port=21
  "Primary Leg Roll [rad, rad/s]" : Outport  Port=22
  "Secondary Leg Roll [rad, rad/s]" : Outport  Port=23
  wires:
  Unit Delay/1 -> ToggleRightLeftLeg/2(previous_right_left)
  ToggleRightLeftLeg/1(right_left) -> Unit Delay/1, Manual Switch/1
  Select Leg/1 -> Manual Switch/2
  R Leg w [m]/1 -> Bus Creator1/10, Bus Creator/3
  R Leg Angle [rad rad/s]/1 -> Bus Creator1/8, Bus Creator/1
  R Leg Length [m m/s]/1 -> Bus Creator1/9, Bus Creator/2
  Bus Creator/1 -> Switch6/1
  Bus Creator1/1 -> Switch6/3
  R Back Joint [rad rad/s]/1 -> Bus Creator1/11, Bus Creator/4
  R Back Gear [rad rad/s]/1 -> Bus Creator1/12, Bus Creator/5
  R Front Joint [rad rad/s]/1 -> Bus Creator1/13, Bus Creator/6
  R Front Gear [rad rad/s]/1 -> Bus Creator1/14, Bus Creator/7
  L Leg Angle [rad rad/s]/1 -> Bus Creator1/1, Bus Creator/8
  L Leg Length [m m/s]/1 -> Bus Creator1/2, Bus Creator/9
  L Leg w [m]/1 -> Bus Creator1/3, Bus Creator/10
  L Back Joint [rad rad/s]/1 -> Bus Creator1/4, Bus Creator/11
  L Back Gear [rad rad/s]/1 -> Bus Creator1/5, Bus Creator/12
  L Front Joint [rad rad/s]/1 -> Bus Creator/13, Bus Creator1/6
  L Front Gear [rad rad/s]/1 -> Bus Creator1/7, Bus Creator/14
  Primary Force/Position Control [1/0]/1 -> Bus Creator1/18, Bus Creator/15
  Primary Back/Front SEA Torque [Nm Nm]/1 -> Bus Creator1/19, Bus Creator/16
  Primary Back/Front Motor Torque [Nm Nm]/1 -> Bus Creator1/20, Bus Creator/17
  Secondary Force/Position Control [1/0]/1 -> Bus Creator1/15, Bus Creator/18
  Secondary Back/Front SEA Torque [Nm Nm]/1 -> Bus Creator1/16, Bus Creator/19
  Secondary Back/Front Motor Torque [Nm Nm]/1 -> Bus Creator1/17, Bus Creator/20
  Switch6/1 -> Bus Selector/1
  Bus Selector/1 -> Primary Leg Angle [rad rad/s]/1  "<signal1>"
  Bus Selector/2 -> Primary Leg Length [m m/s]/1  "<signal2>"
  Bus Selector/3 -> Primary Leg w [m]/1  "<signal3>"
  Bus Selector/4 -> Primary Back Joint [rad rad/s]/1  "<signal4>"
  Bus Selector/5 -> Primary Back Gear [rad rad/s]/1  "<signal5>"
  Bus Selector/6 -> Primary Front Joint [rad rad/s]/1  "<signal6>"
  Bus Selector/7 -> Primary Front Gear [rad rad/s]/1  "<signal7>"
  Bus Selector/8 -> Secondary Leg Angle [rad rad/s]/1  "<signal8>"
  Bus Selector/9 -> Secondary Leg Length [rad rad/s]/1  "<signal9>"
  Bus Selector/10 -> Secondary Leg w [m]/1  "<signal10>"
  Bus Selector/11 -> Secondary Back Joint [rad rad/s]/1  "<signal11>"
  Bus Selector/12 -> Secondary Back Gear [rad rad/s]/1  "<signal12>"
  Bus Selector/13 -> Secondary Front Joint [rad rad/s]/1  "<signal13>"
  Bus Selector/14 -> Secondary Front Gear [rad rad/s]/1  "<signal14>"
  Bus Selector/15 -> R Force/Position Control [1/0]/1  "<signal15>"
  Bus Selector/16 -> R Back/Front SEA Torque [Nm Nm]/1  "<signal16>"
  Bus Selector/17 -> R Back/Front Motor Torque [Nm Nm]/1  "<signal17>"
  Bus Selector/18 -> L Force/Position Control [1/0]/1  "<signal18>"
  Bus Selector/19 -> L Back/Front SEA Torque [Nm Nm]/1  "<signal19>"
  Bus Selector/20 -> L Back/Front Motor Torque [Nm Nm]/1  "<signal20>"
  "Right Leg Roll [rad, rad/s]"/1 -> Bus Creator1/22, Bus Creator/21
  "Left Leg Roll [rad, rad/s]"/1 -> Bus Creator1/21, Bus Creator/22
  Bus Selector/21 -> "Primary Leg Roll [rad, rad/s]"/1  "<signal21>"
  Bus Selector/22 -> "Secondary Leg Roll [rad, rad/s]"/1  "<signal22>"
  Manual Switch/1 -> Right Left Primary/1, Right/Left Primary [1/0]/1, Switch6/2
  System Time [s]/1 -> ToggleRightLeftLeg/3(time_sim), Sum5/2, Enabled Subsystem/1(In1)
  Entering Stance [1/0]/1 -> Enabled Subsystem/Enable, ToggleRightLeftLeg/1(toggle)
  Enabled Subsystem/1(Out1) -> Sum5/1
  Sum5/1 -> Right Left Primary/2

== system atrias_original/control/RC control/Recursive Moving Average ==
  dx [m/s] : Inport
  Delay : Delay  DelayLength=rc.dx_avg_samples  InitialCondition=0  UseCircularBuffer=on  SampleTime=sample_time
  Gain : Gain  Gain=1/(rc.dx_avg_samples)
  Sum : Sum  Inputs=-++
  Unit Delay : UnitDelay  SampleTime=sample_time
  dx_avg [m/s] : Outport
  wires:
  dx [m/s]/1 -> Delay/1, Sum/2
  Sum/1 -> Gain/1, Unit Delay/1
  Delay/1 -> Sum/1
  Gain/1 -> dx_avg [m/s]/1
  Unit Delay/1 -> Sum/3

== system atrias_original/control/RC control/Simbicon leg placcement ==
  Ts [s] : Inport
  dx_des [m/s] : Inport  Port=2
  Foot2CoM : Inport  Port=3
  dx_avg [m/s] : Inport  Port=4
  k_placement : Inport  Port=5
  Cd : Inport  Port=6
  Gain1 : Gain  Gain=0.5
  Mux : Mux  Inputs=2
  Mux1 : Mux  Inputs=2
  Product : Product
  Product1 : Product
  Product2 : Product
  Sum : Sum  Inputs=++-
  Sum2 : Sum  Inputs=-+|
  Ts_saturation : Saturate  UpperLimit=inf  LowerLimit=0.2
      settings: AttributesFormatString=Hi: %<UpperLimit>\nLo: %<LowerLimit>
  d : Scope
  d1 : Scope
  dx : Scope
  dx Saturation : Saturate  UpperLimit=rc.desired_xd  LowerLimit=0
      settings: AttributesFormatString=Hi: %<UpperLimit>\nLo: %<LowerLimit>
  gain_ff : Gain  Gain=rc.gain_ff
  inputs : Scope  NumInputPorts=3
  ts : Scope
  x Saturation : Saturate  UpperLimit=rc.x_limit  LowerLimit=-rc.x_limit
      settings: AttributesFormatString=Hi: %<UpperLimit>\nLo: %<LowerLimit>
  xd_desired : Scope
  desired_footsstep : Outport
  desired_speed : Outport  Port=2
  wires:
  Sum2/1 -> Product1/1
  dx_avg [m/s]/1 -> Mux/1, Mux1/1, Product/2, Sum2/1
  dx_des [m/s]/1 -> desired_speed/1, Mux1/2, Mux/2, Sum2/2
  Product/1 -> Gain1/1
  Ts [s]/1 -> Ts_saturation/1
  Ts_saturation/1 -> ts/1, gain_ff/1
  gain_ff/1 -> Product/1
  Foot2CoM/1 -> Product2/1, d/1
  Gain1/1 -> inputs/2, Sum/2
  Product2/1 -> inputs/1, Sum/1
  Product1/1 -> inputs/3, Sum/3
  Sum/1 -> x Saturation/1
  x Saturation/1 -> d1/1, desired_footsstep/1
  k_placement/1 -> Product1/2
  Cd/1 -> Product2/2
  Mux/1 -> dx/1
  Mux1/1 -> xd_desired/1
